simulink model "CSEI_tau_ellipse"  (R2015a)
settings: Solver=ode4  StartTime=0.0  StopTime=300  FixedStep=0.01  RelTol=1e-3
libraries: simulink x1
settings Model: CovSFcnEnable=off  Creator=rskjetne  LastModifiedBy=MCLab
settings DebuggingCC: UnderspecifiedInitializationDetection=Classic  MergeDetectMultiDrivingBlocksExec=none  SolverPrmCheckMsg=warning
settings RTWCC: SystemTargetFile=NIVeriStand_VxWorks.tlc  TemplateMakefile=NIVeriStand_VxWorks.tmf  Description=NI VeriStand VxWorks Real-Time Target for Release 2007b or later
settings STFCustomTargetCC: GenerateSampleERTMain=off  GeneratePreprocessorConditionals=Disable all  ERTCustomFileBanners=off  MatFileLogging=on  SupportNonInlinedSFcns=on  SupportVariableSizeSignals=off  MATLABClassNameForMDSCustomization=Simulink.SoftwareTarget.TargetSpecificTriggerConfigurationBase  GRTInterface=on  SystemTargetFile=NIVeriStand_VxWorks.tlc

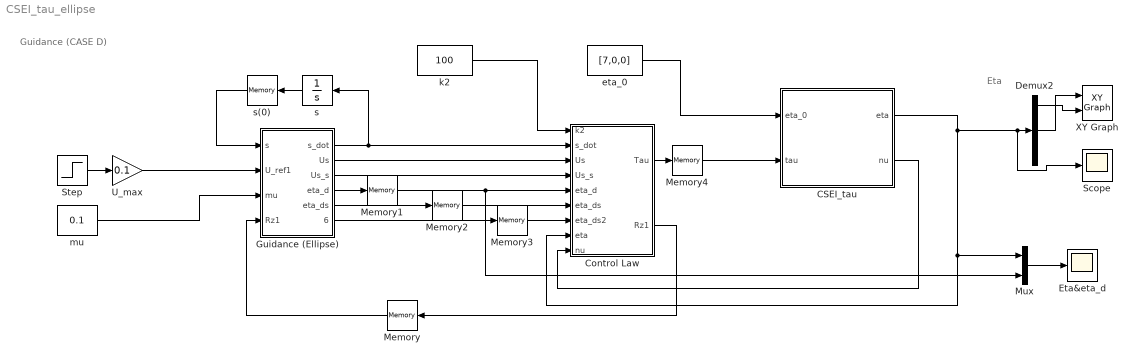
== system CSEI_tau_ellipse ==
  note: Guidance (CASE D)
  note: Eta
  CSEI_tau : Subsystem
  Control Law : MATLAB Function  TreatAsAtomicUnit=on
  Demux2 : Demux  Outputs=3
  Eta&eta_d : Scope
      settings: YMin=-4  YMax=11
  Guidance (Ellipse) : MATLAB Function  TreatAsAtomicUnit=on
  Memory{,1..4} (5 alike) : Memory  X0=[0;0;0]
  Mux : Mux  Inputs=2
  Scope : Scope
      settings: YMin=-4  YMax=12
  Step : Step  Time=2000  Before=1  After=-1  SampleTime=0
  U_max : Gain  Gain=0.1
  XY Graph : simulink/Sinks/XY Graph  xmin=-15  xmax=15  ymin=-15  ymax=15  st=-1
  eta_0 : Constant  Value=[7,0,0]
  k2 : Constant  Value=100
  mu : Constant  Value=0.1
  s : Integrator
  s(0) : Memory
  wires:
  eta_0/1 -> CSEI_tau/1(eta_0)
  Demux2/2 -> XY Graph/1
  Demux2/1 -> XY Graph/2
  Control Law/1(Tau) -> Memory4/1
  CSEI_tau/1(eta) -> Control Law/8(eta), Mux/1, Scope/1, Demux2/1
  CSEI_tau/2(nu) -> Control Law/9(nu)
  Step/1 -> U_max/1
  U_max/1 -> Guidance (Ellipse)/2(U_ref1)
  mu/1 -> Guidance (Ellipse)/3(mu)
  Guidance (Ellipse)/1(s_dot) -> s/1, Control Law/2(s_dot)
  s/1 -> s(0)/1
  Guidance (Ellipse)/4(eta_d) -> Memory1/1
  Guidance (Ellipse)/5(eta_ds) -> Memory2/1
  Control Law/2(Rz1) -> Memory/1
  Memory/1 -> Guidance (Ellipse)/4(Rz1)
  Guidance (Ellipse)/2(Us) -> Control Law/3(Us)
  s(0)/1 -> Guidance (Ellipse)/1(s)
  Guidance (Ellipse)/3(Us_s) -> Control Law/4(Us_s)
  Guidance (Ellipse)/6(eta_ds2) -> Memory3/1
  Memory1/1 -> Mux/2, Control Law/5(eta_d)
  Memory2/1 -> Control Law/6(eta_ds)
  Memory3/1 -> Control Law/7(eta_ds2)
  Memory4/1 -> CSEI_tau/2(tau)
  k2/1 -> Control Law/1(k2)
  Mux/1 -> Eta&eta_d/1

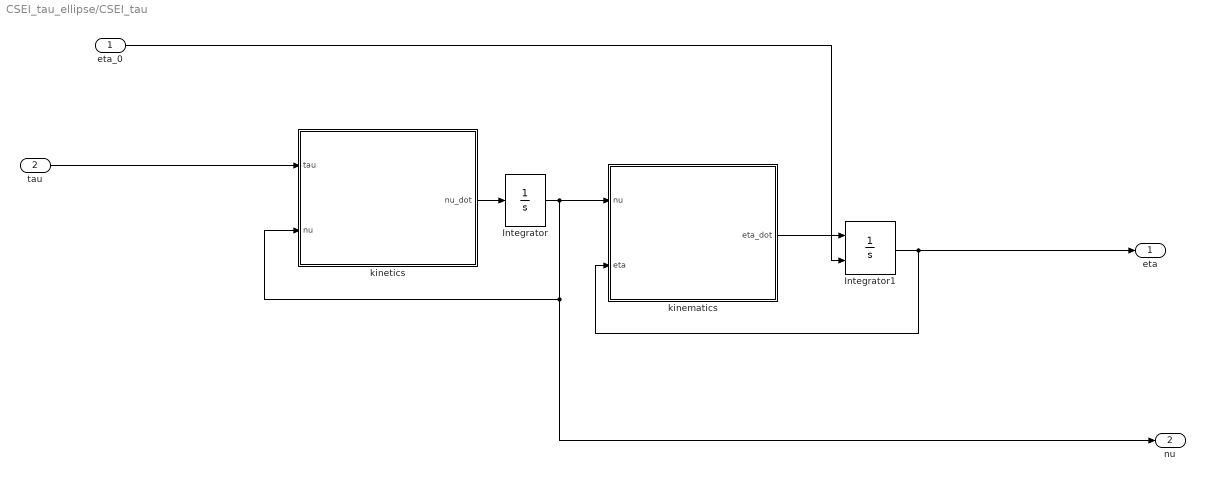
== system CSEI_tau_ellipse/CSEI_tau ==
  eta_0 : Inport
  tau : Inport  Port=2
  Integrator : Integrator  InitialCondition=[0 0 0]'
  Integrator1 : Integrator  InitialConditionSource=external  InitialCondition=[0 0 0]'
  kinematics : MATLAB Function  TreatAsAtomicUnit=on
  kinetics : MATLAB Function  TreatAsAtomicUnit=on
  eta : Outport
  nu : Outport  Port=2
  wires:
  kinetics/1(nu_dot) -> Integrator/1
  Integrator/1 -> nu/1, kinetics/2(nu), kinematics/1(nu)
  kinematics/1(eta_dot) -> Integrator1/1
  Integrator1/1 -> eta/1, kinematics/2(eta)
  eta_0/1 -> Integrator1/2
  tau/1 -> kinetics/1(tau)

== matlab function CSEI_tau_ellipse/CSEI_tau/kinematics ==
  data: nu input; eta_dot output; eta input
function eta_dot = CSE1_eta_dot(nu,eta)

psi = eta(3);

J = [cos(psi) -sin(psi) 0
     sin(psi) cos(psi)  0
     0        0         1];

eta_dot = J*nu;

== matlab function CSEI_tau_ellipse/CSEI_tau/kinetics ==
  data: tau input; nu_dot output; nu input
function nu_dot = CSE1_nu_dot(tau,nu)

u   = nu(1);
v   = nu(2);
r   = nu(3);

tau = [tau(1);tau(2);tau(3)];
%% MATRICES

m    = 14.79;   I_z  =  1.7600;   x_g = 0.0375;       % x_g  =  0.0460; % Table B.1


%% Added mass
X_ud  =     -2.0;											% Table B.1
					Y_vd =     -1.0;	N_vd =    -0.0;		% Table B.1 guestimate
					Y_rd =      -0.0;	N_rd =    -1.0;		% Table B.1

%% Total mass matrix
m_11 = m-X_ud;
m_22 = m-Y_vd;
m_23 = m*x_g-Y_rd;
m_32 = m*x_g-N_vd;
m_33 = I_z-N_rd;

M    = [m_11 0    0
        0    m_22 m_23
        0    m_32 m_33];
	
%% Damping coefficients
% Comments at the end of the lines indicate the old values used.
X_u		= -0.6555;		X_v		= 0;
X_uu 	= 0.3545;		X_vv	= -2.443;
X_uuu 	= -3.787;		X_vvv	= 0;

						Y_v		= -1.33; 			Y_r		= -7.250; % Y_r
						Y_vv	= -2.776;			Y_rr	= -3.450; % Y_rr
						Y_vvv	= -64.91;			Y_rrr	= 0;
						
						Y_rv	= -0.805;			Y_vr	= -0.845; % Y_rv, Y_vr

						N_v		= 0;				N_r		= -1.900; % N_r
						N_vv	= -0.2088;			N_rr	= -0.750; % N_rr
						N_vvv	= 0;				N_rrr	= 0;
						
						N_rv	= 0.130;			N_vr	= 0.080; % N_rv, N_vr

%% Correolis matrix
c_13 = -(m-Y_vd)*v-(m*x_g-Y_rd)*r;
c_23 = (m-X_ud)*u;
C    = [0     0     c_13
        0     0     c_23
        -c_13 -c_23 0   ];

%% Assembly of the damping matrix
d_11 = -X_u - X_uu*u - X_uuu*u^2;
d_22 = -Y_v - Y_vv*v - Y_vvv*v^2 - Y_rv*abs(r);
d_33 = -N_r - N_rr*abs(r) - N_rrr*r^2 - N_vr*abs(v); % using abs(r)

d_12 = -X_v - X_vv*v - X_vvv*v^2;
d_23 = -Y_r - Y_rr*abs(r) - Y_rrr*r^2 - Y_vr*abs(v);
d_32 = -N_v - N_vv*v - N_vvv*v^2 - N_rv*abs(r);

D    = [d_11 d_12 0
        0    d_22 d_23
        0    d_32 d_33];



%% CALCULATION
nu_dot = M\(tau-(C+D)*nu);

== matlab function CSEI_tau_ellipse/Control Law ==
  data: k2 input; s_dot input; Us input; Us_s input; eta_d input; eta_ds input; eta_ds2 input; eta input; Tau output; Rz1 output; nu input
function [Tau,Rz1] = fcn(k2,s_dot,Us,Us_s,eta_d,eta_ds,eta_ds2,eta,nu)

%% ROTATION MATRICES

psi = 0;
Tau = [0;0;0];
psi = eta(3);   % psi : yaw angle
r = nu(3);      % r : yaw rate
u = nu(1);      % u : surge velocity
v = nu(2);      % v : sway velocity


R = [ cos(psi) , -sin(psi) , 0 ;
      sin(psi) , cos(psi)  , 0 ;
      0            0         1 ] ;

S = [ 0 , -r , 0 ;
       r , 0 , 0 ;
       0 , 0 , 0 ];

   
%% MASS MATRIX (from CSEI_tau)

m    = 14.79;   I_z  =  1.7600;   x_g = 0.0375;       % x_g  =  0.0460; % Table B.1

% Added mass
X_ud  =     -2.0;											% Table B.1
					Y_vd =     -1.0;	N_vd =    -0.0;		% Table B.1 guestimate
					Y_rd =      -0.0;	N_rd =    -1.0;		% Table B.1
                    
% Total mass matrix
m_11 = m-X_ud;
m_22 = m-Y_vd;
m_23 = m*x_g-Y_rd;
m_32 = m*x_g-N_vd;
m_33 = I_z-N_rd;

M    = [m_11 0    0
        0    m_22 m_23
        0    m_32 m_33];
	
%% DAMPING MATRIX (from CSEI_tau)
X_u		= -0.6555;		X_v		= 0;
X_uu 	= 0.3545;		X_vv	= -2.443;
X_uuu 	= -3.787;		X_vvv	= 0;

						Y_v		= -1.33; 			Y_r		= -7.250; % Y_r
						Y_vv	= -2.776;			Y_rr	= -3.450; % Y_rr
						Y_vvv	= -64.91;			Y_rrr	= 0;
						
						Y_rv	= -0.805;			Y_vr	= -0.845; % Y_rv, Y_vr

						N_v		= 0;				N_r		= -1.900; % N_r
						N_vv	= -0.2088;			N_rr	= -0.750; % N_rr
						N_vvv	= 0;				N_rrr	= 0;
						
						N_rv	= 0.130;			N_vr	= 0.080; % N_rv, N_vr

% Assembly of the damping matrix
d_11 = -X_u - X_uu*u - X_uuu*u^2;
d_22 = -Y_v - Y_vv*v - Y_vvv*v^2 - Y_rv*abs(r);
d_33 = -N_r - N_rr*abs(r) - N_rrr*r^2 - N_vr*abs(v); % using abs(r)

d_12 = -X_v - X_vv*v - X_vvv*v^2;
d_23 = -Y_r - Y_rr*abs(r) - Y_rrr*r^2 - Y_vr*abs(v);
d_32 = -N_v - N_vv*v - N_vvv*v^2 - N_rv*abs(r);

D    = [d_11 d_12 0
        0    d_22 d_23
        0    d_32 d_33];


%% CASE D


K_p = diag([0.2,0.2,0.1]);          % Kp (tuning)
K2 = k2 * diag([1,1,1]);           % K2 (tuning)

z1 = R'*(eta-eta_d);                % z1
alpha1 = -K_p*z1 + R'*eta_ds*Us ;   % alpha1
Rz1 = R*z1 ;                        % R*z1

z1_dot = S'*z1+nu-R'*eta_ds*s_dot;  % z1_dot
a1_dot = -K_p*z1_dot+(R*S)'*eta_ds*Us + R'*(eta_ds2*Us+eta_ds*Us_s)*s_dot;    % alpha1_dot

z2 = nu - alpha1 ;                  % z2

Tau = D*nu  +   M*a1_dot - K2*z2 - z1 ;     % Tau



end

== matlab function CSEI_tau_ellipse/Guidance (Ellipse) ==
  data: s input; s_dot output; Us output; U_ref1 input; mu input; Rz1 input; Us_s output; eta_d output; eta_ds output; eta_ds2 output
function [s_dot,Us,Us_s,eta_d,eta_ds,eta_ds2] = f(s,U_ref1,mu,Rz1)

%% Ellipse Kinematics

eta_d = [0;0;0];
eta_ds = [0;0;0];
eta_ds2 = [0;0;0];

cx = 6;
cy = 0;
rx = 5;
ry = 3;

x_d = cx+rx*cos(s);
y_d = cy+ry*sin(s);

x_ds = -rx*sin(s);
y_ds = ry*cos(s);

x_ds2 = -rx*cos(s);
y_ds2 = -ry*sin(s);

x_ds3 = rx*sin(s);
y_ds3 = -ry*cos(s);

psi_d = atan2(y_ds,x_ds);
psi_ds = (-y_ds*x_ds+x_ds*y_ds2)/(x_ds^2+y_ds^2);
psi_ds2 = ( (-y_ds*x_ds3+x_ds*y_ds3)*(x_ds^2+y_ds^2) - (-y_ds*x_ds2+x_ds*y_ds2)*(2*x_ds2*x_ds+2*y_ds2*y_ds) )/(x_ds^2+y_ds^2)^2;

eta_d = [x_d;y_d;psi_d] ;
eta_ds = [x_ds;y_ds;psi_ds];
eta_ds2 = [x_ds2;y_ds2;psi_ds2];

Us = U_ref1 / (x_ds^2+y_ds^2)^(1/2);
Us_s = U_ref1 * (x_ds*x_ds2 + y_ds*y_ds2) / (x_ds^2+y_ds^2)^(3/2);


%% Update Law

V1 = - eta_ds'*Rz1 ;
s_dot = Us - mu*V1/norm(eta_ds);


end
